simulink model "car"  (Simulink 8.0)
settings: Solver=ode45  StartTime=0.0  StopTime=30.0  RelTol=1e-3
model workspace (MAT data in the model file):
  Vup = [10  30  50  1000000; 10  30  50  1000000; 15  30  50  1000000; 23  41  60  1000000; 40  70  100  1000000; 40  70  100  1000000]
  Vdown = [0  5  20  35; 0  5  20  35; 0  5  25  40; 0  5  30  50; 0  30  50  80; 0  30  50  80]
  THup = [0; 25; 35; 50; 90; 100]
  THdown = [0; 5; 40; 50; 90; 100]
  TH = [0; 20; 30; 40; 50; 60; 70; 80; 90; 100]
  Te = [-40  -44  -49  -53  -57  -61  -65  -70  -74  -78  -82; 215  117  85  66  44  29  10  -2  -13  -22  -32; 245  208  178  148  122  104  85  66  48  33  18; 264  260  241  219  193  167  152  133  119  96  85; 264  279  282  275  260  238  223  208  189  171  152; 267  290  293  297  290  275  260  256  234  212  193; 267  297  305  305  305  301  293  282  267  249  226; 267  301  308  312  319  323  319  316  297  279  253; 267  301  312  319  327  327  327  327  312  293  267; 267  301  312  319  327  334  334  334  319  305  275]
  Rw = 1
  Qt = [2.232; 2.075; 1.975; 1.846; 1.72; 1.564; 1.409; 1.254; 1.096; 1.08; 1.061; 1.043; 1.028; 1.012; 1.002; 1.002; 1.001; 0.998; 0.999; 1.001; 1.002]
  Qn = [0; 0.1; 0.2; 0.3; 0.4; 0.5; 0.6; 0.7; 0.8; 0.81; 0.82; 0.83; 0.84; 0.85; 0.86; 0.87; 0.88; 0.89; 0.9; 0.92; 0.94]
  Qfd = 3.23
  Ne = [800 1200 1600 2000 2400 2800 3200 3600 4000 4400 4800]
  K = [137.465208994; 137.065019157; 135.864449646; 135.664354728; 137.565256453; 140.366585312; 145.268910814; 152.872517717; 162.9773111; 164.27792807; 166.178829795; 167.979684062; 170.080680706; 172.781962105; 175.383196045; 179.585189333; 183.587087703; 189.890077635; 197.693779455; 215.902417037; 244.515990379]
  Iv = 12.0941478573
  Ie = 0.0219914882836
  F = 40
  Cd : num (value not decoded)
undefined symbols (not defined in the file): sigbuilder_block
settings Model: Creator=oqaqish  LastModifiedBy=ZhouHaoyu
settings DataIOCC: SignalLoggingSaveFormat=ModelDataLogs  SignalLoggingName=sigsOut
settings OptimizationCC: InlineInvariantSignals=on  InitFltsAndDblsToZero=on
settings DebuggingCC: SaveWithParameterizedLinksMsg=none  CheckExecutionContextPreStartOutputMsg=on  CheckExecutionContextRuntimeOutputMsg=on  SignalResolutionControl=TryResolveAllWithWarning  SolverPrmCheckMsg=none  MultiTaskDSMMsg=warning  MultiTaskCondExecSysMsg=none  FcnCallInpInsideContextMsg=UseLocalSettings  StrictBusMsg=None
settings HardwareCC: TargetUnknown=on
settings RTWCC: IncludeERTFirstTime=on
settings GRTTargetCC: TargetFcnLib=ansi_tfl_tmw.mat  ModelReferenceCompliant=off  CombineOutputUpdateFcns=off  MatFileLogging=off  GRTInterface=on

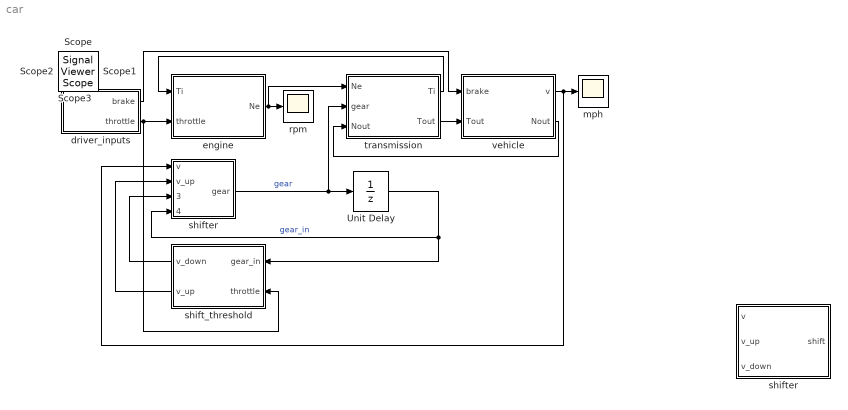
== system car ==
  Unit Delay : UnitDelay  InitialCondition=1  SampleTime=0.05
      settings: AttributesFormatString=Ts = %<SampleTime>\n
  driver_inputs : Subsystem  Tag=STV Subsys  LoadFcn=sigbuilder_block('load');  StartFcn=sigbuilder_block('start');  StopFcn=sigbuilder_block('stop');  ClipboardFcn=sigbuilder_block('clipboard');  mask(Sigbuilder block){}
      mask help: Sigbuilder GUI
      mask init:
      | tuvar = sigbuilder_block('maskInit');
      settings: CopyFcn=sigbuilder_block('copy');  DeleteFcn=sigbuilder_block('delete');  ModelCloseFcn=sigbuilder_block('modelClose');  PreSaveFcn=sigbuilder_block('preSave');  PauseFcn=sigbuilder_block('pause')  ContinueFcn=sigbuilder_block('continue')  NameChangeFcn=sigbuilder_block('namechange');  OpenFcn=sigbuilder_block('open',[113.25 99.75 519.75 399.75 ]);  CloseFcn=sigbuilder_block('close');
      mask Display: plot(0,0,100,100,[10,10,40,40,10],[80,20,20,80,80],[40,10],[50,50], [40,27,10],[65,72,56],[40,25,25,10],[28,28,43,43]);
  engine : Subsystem
  mph : Scope
      settings: TimeRange=30  YMin=0  YMax=140
  rpm : Scope
      settings: TimeRange=30  YMin=1000  YMax=6000
  shift_threshold : Subsystem
  shifter : Subsystem
  "shifter " : Stateflow chart  TreatAsAtomicUnit=on
  transmission : Subsystem
  vehicle : Subsystem
  Scope{,1..3} (4 alike) : SignalViewerScope  IOType=viewer  RefreshTime=0.035000
      Scope2 settings: SaveName=ScopeData2
      Scope3 settings: SaveName=ScopeData3
  wires:
  driver_inputs/2(throttle) -> shift_threshold/2(throttle), engine/2(throttle)
  engine/1(Ne) -> transmission/1(Ne), rpm/1
  transmission/1(Ti) -> engine/1(Ti)
  driver_inputs/1(brake) -> vehicle/1(brake)
  transmission/2(Tout) -> vehicle/2(Tout)
  Unit Delay/1 -> "shifter "/4(gear_in), shift_threshold/1(gear_in)  "gear_in"
  vehicle/2(Nout) -> transmission/3(Nout)
  vehicle/1(v) -> "shifter "/1(v), mph/1
  "shifter "/1(gear) -> transmission/2(gear), Unit Delay/1  "gear"
  shift_threshold/1(v_down) -> "shifter "/3(v_down)
  shift_threshold/2(v_up) -> "shifter "/2(v_up)

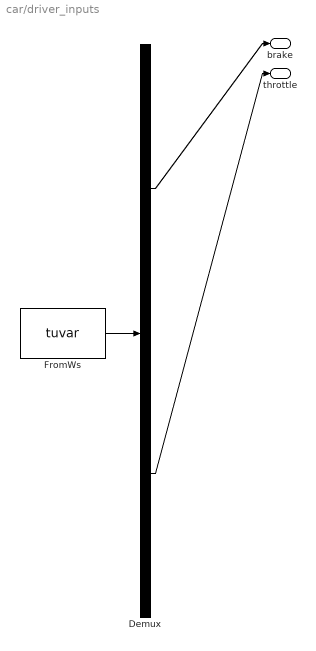
== system car/driver_inputs ==
  Demux : Demux  Tag=STV Demux  Outputs=2
  FromWs : FromWorkspace  Tag=STV FromWs  VariableName=tuvar  SampleTime=0  SigBuilderData=DataTag1  VnvData=DataTag2
      SigBuilderData=|
      | dataSet.timeRange = [0 50]
      | dataSet.name = 'Passing Manuver'
      | sbobj.Groups.Name = 'Passing Manuver'
      | sbobj.Groups.Signals(1).Name = 'brake'
      | sbobj.Groups.Signals(1).XData = [0 50]
      | sbobj.Groups.Signals(1).YData = [0 0]
      | sbobj.Groups.Signals(2).Name = 'throttle'
      | sbobj.Groups.Signals(2).XData = [0 15 15 50]
      | sbobj.Groups.Signals(2).YData = [60 40 100 60]
      | sbobj.Groups.TimeRange = [0 50]
  brake : Outport  Tag=STV Outport
  throttle : Outport  Tag=STV Outport  Port=2
  wires:
  Demux/2 -> throttle/1
  Demux/1 -> brake/1
  FromWs/1 -> Demux/1

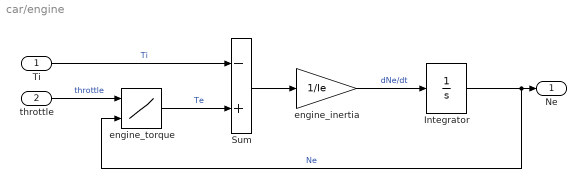
== system car/engine ==
  Ti : Inport
  throttle : Inport  Port=2
  Integrator : Integrator  InitialCondition=1000  LimitOutput=on  UpperSaturationLimit=6000  LowerSaturationLimit=600  ZeroCross=off
      settings: AttributesFormatString="Ne0 = %<InitialCondition>\\n%<LowerSaturationLimit> <= Ne <=  %<UpperSaturationLimit>\\n\\n"
  Sum : Sum  Inputs=-+  SaturateOnIntegerOverflow=on  InputSameDT=on  OutDataTypeStr=Inherit: Same as first input
  engine_inertia : Gain  Gain=1/Ie  SaturateOnIntegerOverflow=on  OutDataTypeStr=Inherit: Same as input  ParamDataTypeStr=Inherit: Same as input
  engine_torque : Lookup2D  RowIndex=TH  ColumnIndex=Ne  Table=Te  SaturateOnIntegerOverflow=on
  Ne : Outport
  wires:
  Sum/1 -> engine_inertia/1
  throttle/1 -> engine_torque/1  "throttle"
  engine_torque/1 -> Sum/2  "Te"
  Ti/1 -> Sum/1  "Ti"
  Integrator/1 -> Ne/1, engine_torque/2  "Ne"
  engine_inertia/1 -> Integrator/1  "dNe/dt"

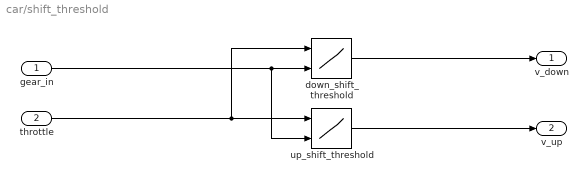
== system car/shift_threshold ==
  gear_in : Inport
  throttle : Inport  Port=2
  down_shift_threshold : Lookup2D  RowIndex=THdown  ColumnIndex=[1:4]  Table=Vdown  InputSameDT=on
  up_shift_threshold : Lookup2D  RowIndex=THup  ColumnIndex=[1:4]  Table=Vup  InputSameDT=on
  v_down : Outport
  v_up : Outport  Port=2
  wires:
  up_shift_threshold/1 -> v_up/1
  down_shift_threshold/1 -> v_down/1
  throttle/1 -> up_shift_threshold/1, down_shift_threshold/1
  gear_in/1 -> up_shift_threshold/2, down_shift_threshold/2

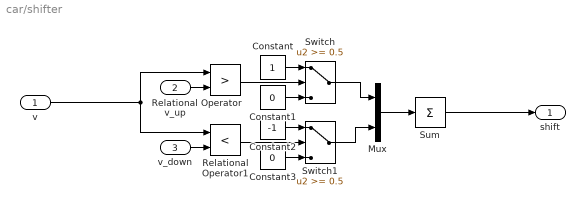
== system car/shifter ==
  v : Inport  SampleTime=0.05
  v_up : Inport  Port=2  SampleTime=0.05
  v_down : Inport  Port=3  SampleTime=0.05
  Constant : Constant
  Constant1 : Constant  Value=0
  Constant2 : Constant  Value=-1
  Constant3 : Constant  Value=0
  Mux : Mux  Inputs=2
  Relational Operator : RelationalOperator  Operator=>
  Relational Operator1 : RelationalOperator  Operator=<
  Sum : Sum  Inputs=1  SaturateOnIntegerOverflow=on
  Switch : Switch  Threshold=0.5  SaturateOnIntegerOverflow=on
      settings: AttributesFormatString=T = %<Threshold>\n
  Switch1 : Switch  Threshold=0.5  SaturateOnIntegerOverflow=on
      settings: AttributesFormatString=T = %<Threshold>\n
  shift : Outport
  wires:
  v_up/1 -> Relational Operator/2
  v_down/1 -> Relational Operator1/2
  Relational Operator/1 -> Switch/2
  Switch/1 -> Mux/1
  Mux/1 -> Sum/1
  v/1 -> Relational Operator/1, Relational Operator1/1
  Constant/1 -> Switch/1
  Constant1/1 -> Switch/3
  Relational Operator1/1 -> Switch1/2
  Constant2/1 -> Switch1/1
  Constant3/1 -> Switch1/3
  Switch1/1 -> Mux/2
  Sum/1 -> shift/1

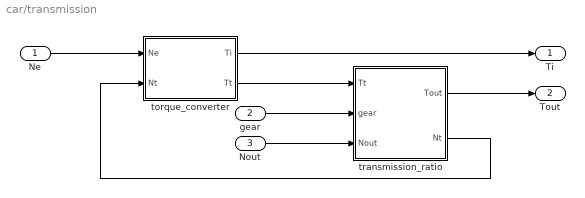
== system car/transmission ==
  Ne : Inport
  gear : Inport  Port=2
  Nout : Inport  Port=3
  torque_converter : Subsystem
  transmission_ratio : Subsystem
  Ti : Outport  InitialOutput=0
  Tout : Outport  Port=2  InitialOutput=0
  wires:
  transmission_ratio/2(Nt) -> torque_converter/2(Nt)
  Ne/1 -> torque_converter/1(Ne)
  gear/1 -> transmission_ratio/2(gear)
  Nout/1 -> transmission_ratio/3(Nout)
  transmission_ratio/1(Tout) -> Tout/1
  torque_converter/2(Tt) -> transmission_ratio/1(Tt)
  torque_converter/1(Ti) -> Ti/1

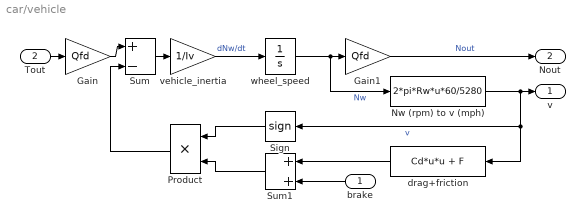
== system car/vehicle ==
  brake : Inport
  Tout : Inport  Port=2
  Gain : Gain  Gain=Qfd  SaturateOnIntegerOverflow=on  OutDataTypeStr=Inherit: Same as input  ParamDataTypeStr=Inherit: Same as input
  Gain1 : Gain  Gain=Qfd  SaturateOnIntegerOverflow=on  OutDataTypeStr=Inherit: Same as input  ParamDataTypeStr=Inherit: Same as input
  Nw (rpm) to v (mph) : Fcn  Expr=2*pi*Rw*u*60/5280
  Product : Product  SaturateOnIntegerOverflow=on  OutDataTypeStr=Inherit: Same as first input
  Sign : Signum
  Sum : Sum  Inputs=|+-  SaturateOnIntegerOverflow=on
  Sum1 : Sum  SaturateOnIntegerOverflow=on
  drag+friction : Fcn  Expr=Cd*u*u + F
  vehicle_inertia : Gain  Gain=1/Iv  SaturateOnIntegerOverflow=on  OutDataTypeStr=Inherit: Same as input  ParamDataTypeStr=Inherit: Same as input
  wheel_speed : Integrator
      settings: AttributesFormatString=Nw0 = %<InitialCondition>\n
  v : Outport
  Nout : Outport  Port=2
  wires:
  Tout/1 -> Gain/1
  Gain/1 -> Sum/1
  Sum/1 -> vehicle_inertia/1
  wheel_speed/1 -> Gain1/1, Nw (rpm) to v (mph)/1  "Nw"
  Gain1/1 -> Nout/1  "Nout"
  Nw (rpm) to v (mph)/1 -> v/1, Sign/1, drag+friction/1  "v"
  vehicle_inertia/1 -> wheel_speed/1  "dNw/dt"
  brake/1 -> Sum1/2
  drag+friction/1 -> Sum1/1
  Sign/1 -> Product/1
  Sum1/1 -> Product/2
  Product/1 -> Sum/2

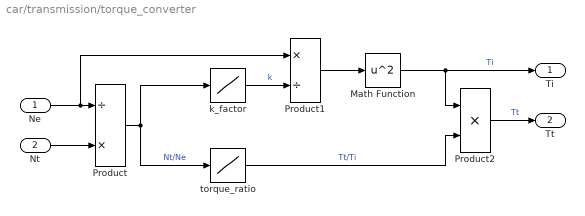
== system car/transmission/torque_converter ==
  Ne : Inport
  Nt : Inport  Port=2
  Math Function : Math  Operator=square  SaturateOnIntegerOverflow=on
  Product : Product  Inputs=/*  SaturateOnIntegerOverflow=on  OutDataTypeStr=Inherit: Same as first input
  Product1 : Product  Inputs=*/  SaturateOnIntegerOverflow=on  OutDataTypeStr=Inherit: Same as first input
  Product2 : Product  Inputs=**  SaturateOnIntegerOverflow=on  OutDataTypeStr=Inherit: Same as first input
  k_factor : Lookup  InputValues=Qn  Table=K  SaturateOnIntegerOverflow=on
  torque_ratio : Lookup  InputValues=Qn  Table=Qt  SaturateOnIntegerOverflow=on
  Ti : Outport
  Tt : Outport  Port=2
  wires:
  Product1/1 -> Math Function/1
  torque_ratio/1 -> Product2/2  "Tt/Ti"
  Math Function/1 -> Product2/1, Ti/1  "Ti"
  k_factor/1 -> Product1/2  "k"
  Product/1 -> k_factor/1, torque_ratio/1  "Nt/Ne"
  Ne/1 -> Product1/1, Product/1
  Product2/1 -> Tt/1  "Tt"
  Nt/1 -> Product/2

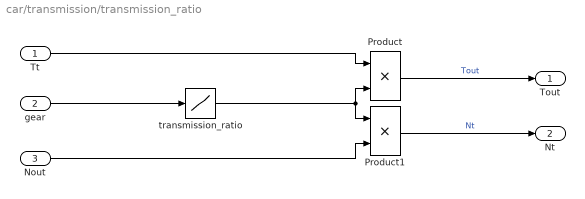
== system car/transmission/transmission_ratio ==
  Tt : Inport
  gear : Inport  Port=2
  Nout : Inport  Port=3
  Product : Product  SaturateOnIntegerOverflow=on  InputSameDT=on  OutDataTypeStr=Inherit: Same as first input
  Product1 : Product  SaturateOnIntegerOverflow=on  InputSameDT=on  OutDataTypeStr=Inherit: Same as first input
  transmission_ratio : Lookup  InputValues=[1, 2, 3, 4]  Table=[2.393, 1.450, 1.000, 0.677]  SaturateOnIntegerOverflow=on
  Tout : Outport  InitialOutput=0
  Nt : Outport  Port=2  InitialOutput=0
  wires:
  gear/1 -> transmission_ratio/1
  Tt/1 -> Product/1
  Product/1 -> Tout/1  "Tout"
  Product1/1 -> Nt/1  "Nt"
  Nout/1 -> Product1/2
  transmission_ratio/1 -> Product1/1, Product/2

== stateflow chart shifter  ==
  state State1
    entry: shift=1;
    gear=shift+gear_in;
  state Start
  state State2
    entry: shift=0;
    gear=shift+gear_in;
  state State3
    entry: shift=-1;
    gear=shift+gear_in;
  (default) -> Start
  Start -> State1 [order 1] : [ v>v_up ]
  Start -> State2 [order 2] : [ v>v_down && v<v_up]
  State1 -> State2 : [ v>v_down && v<v_up]
  State2 -> State1 [order 2] : [ v>v_up ]
  Start -> State3 [order 3] : [ v<v_down ]
  State3 -> State2 : [ v>v_down && v<v_up]
  State2 -> State3 [order 1] : [ v<v_down]
  data: v input double; v_up input double; v_down input double; gear_in input double; gear output double; shift local double
